simulink model "PV_Array_Application_DC_converor"  (Simulink 7.5)
settings: Solver=ode5  StartTime=0.0  StopTime=10.0  FixedStep=0.00001  RelTol=1e-3
libraries: powerlib x9, simulink x6
settings Model: Creator=Leo216  LastModifiedBy=Leo216

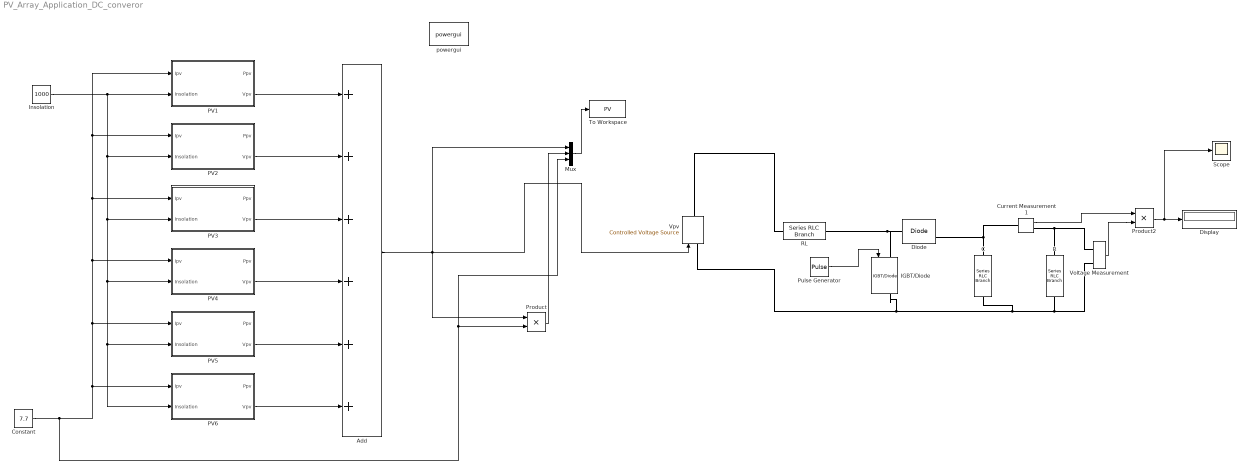
== system PV_Array_Application_DC_converor ==
  Add : Sum  Inputs=++++++  OutDataType=fixdt(1, 16)  OutScaling=2^-10
  C : powerlib/Elements/Series RLC Branch  DialogController=POWERSYS.PowerSysDialog  PhysicalDomain=powersysdomain  SubClassName=unknown  LeftPortType=p1  RightPortType=p1  LConnTagsString=__new0  RConnTagsString=__new0  BranchType=C  Resistance=1  Inductance=1e-3  SetiL0=off  InitialCurrent=0  Capacitance=2000e-6  Setx0=off  InitialVoltage=0  Measurements=None
  Constant : Constant  Value=7.7  OutDataType=fixdt(1, 16)  OutScaling=2^0
  Current Measurement1 : powerlib/Measurements/Current Measurement  DialogController=POWERSYS.PowerSysDialog  SystemSampleTime=-1  PhasorSimulation=off  OutputType=Complex  PSBequivalent=0
  Diode : powerlib/Power Electronics/Diode  DialogController=POWERSYS.PowerSysDialog  SystemSampleTime=-1  Ron=0.001  Lon=0  Vf=0.8  IC=0  UseSnubber=off  Rs=500  Cs=250e-9  Measurements=on
  Display : Display
  IGBT/Diode : powerlib/Power Electronics/IGBT//Diode  DialogController=POWERSYS.PowerSysDialog  SystemSampleTime=-1  Ron=1e-3  Rs=1e5  Cs=inf  Measurements=on
  Insolation : Constant  Value=1000  OutDataType=fixdt(1, 16)  OutScaling=2^0  SampleTime=-1
  Mux : Mux  Inputs=3
  PV1 : Subsystem  mask{Isc=8.4, Voc=39.6/63, Ir=7.7, Vr=31.9/63, Diode=on}
      mask prompts: Isc "Short-circuit current"; Voc "Open-Circuit Voltage"; Ir "Current at Pmax"; Vr "Voltage at Pmax"; Diode "By-pass diode"
      mask init:
      | Ns=round(Voc/0.61);
      | Vt=26e-3
      | G= Isc/1000;
      | Vmpc=Vr/Ns;
      | Vocc=Voc/Ns;
      | Rmpp=Vmpc/Ir;
      | 
      | Rp=100*Vocc/Isc;
      | Vdm=Vocc;
      | 
      | for i=1:10
      |     
      |    Idm=Isc-Ir-Vdm/Rp;
      |    Io=(Isc-Vocc/Rp)/(exp(Vocc/Vt)-1);
      |    Vdm=Vt*log(Idm/Io+1);
      |    Rs=(Vdm-Vmpc)/Ir;
      |    Rd=(Rmpp-Rs)*Rp/(Rp-Rmpp+Rs);
      |    Idm=Vt/Rd;
      |    Rp=Vdm/(Isc-Ir-Idm);
      |    
      | end
      mask Display: image(imread('pv.jpg'))
  PV2 : Subsystem  mask{Isc=8.4, Voc=39.6/63, Ir=7.7, Vr=31.9/63, Diode=on}
      mask prompts: Isc "Short-circuit current"; Voc "Open-Circuit Voltage"; Ir "Current at Pmax"; Vr "Voltage at Pmax"; Diode "By-pass diode"
      mask init: same as PV_Array_Application_DC_converor/PV1
      mask Display: image(imread('pv.jpg'))
  PV3 : Subsystem  mask{Isc=8.4, Voc=39.6/63, Ir=7.7, Vr=31.9/63, Diode=on}
      mask prompts: Isc "Short-circuit current"; Voc "Open-Circuit Voltage"; Ir "Current at Pmax"; Vr "Voltage at Pmax"; Diode "By-pass diode"
      mask init: same as PV_Array_Application_DC_converor/PV1
      mask Display: image(imread('pv.jpg'))
  PV4 : Subsystem  mask{Isc=8.4, Voc=39.6/63, Ir=7.7, Vr=31.9/63, Diode=on}
      mask prompts: Isc "Short-circuit current"; Voc "Open-Circuit Voltage"; Ir "Current at Pmax"; Vr "Voltage at Pmax"; Diode "By-pass diode"
      mask init: same as PV_Array_Application_DC_converor/PV1
      mask Display: image(imread('pv.jpg'))
  PV5 : Subsystem  mask{Isc=8.4, Voc=39.6/63, Ir=7.7, Vr=31.9/63, Diode=on}
      mask prompts: Isc "Short-circuit current"; Voc "Open-Circuit Voltage"; Ir "Current at Pmax"; Vr "Voltage at Pmax"; Diode "By-pass diode"
      mask init: same as PV_Array_Application_DC_converor/PV1
      mask Display: image(imread('pv.jpg'))
  PV6 : Subsystem  mask{Isc=8.4, Voc=39.6/63, Ir=7.7, Vr=31.9/63, Diode=on}
      mask prompts: Isc "Short-circuit current"; Voc "Open-Circuit Voltage"; Ir "Current at Pmax"; Vr "Voltage at Pmax"; Diode "By-pass diode"
      mask init: same as PV_Array_Application_DC_converor/PV1
      mask Display: image(imread('pv.jpg'))
  Product : Product  OutDataType=fixdt(1, 16)  OutScaling=2^0  RndMeth=Zero
  Product2 : Product  OutDataType=fixdt(1, 16)  OutScaling=2^0  RndMeth=Zero
  Pulse Generator : DiscretePulseGenerator  PulseType=Time based  Amplitude=1  Period=.0001  PulseWidth=50  PhaseDelay=0  SampleTime=1
  R : powerlib/Elements/Series RLC Branch  DialogController=POWERSYS.PowerSysDialog  PhysicalDomain=powersysdomain  SubClassName=unknown  LeftPortType=p1  RightPortType=p1  LConnTagsString=__new0  RConnTagsString=__new0  BranchType=R  Resistance=1.576  Inductance=1e-3  SetiL0=off  InitialCurrent=0  Capacitance=1e-6  Setx0=off  InitialVoltage=0  Measurements=None
  RL : powerlib/Elements/Series RLC Branch  DialogController=POWERSYS.PowerSysDialog  PhysicalDomain=powersysdomain  SubClassName=unknown  LeftPortType=p1  RightPortType=p1  LConnTagsString=__new0  RConnTagsString=__new0  BranchType=RL  Resistance=0.005  Inductance=6e-3  SetiL0=off  InitialCurrent=0  Capacitance=1e-6  Setx0=off  InitialVoltage=0  Measurements=None
  Scope : Scope
      settings: YMin=17.075  YMax=17.55
  To Workspace : ToWorkspace  VariableName=PV  SampleTime=-1  SaveFormat=Structure
  Voltage Measurement : powerlib/Measurements/Voltage Measurement  DialogController=POWERSYS.PowerSysDialog  SystemSampleTime=-1  PhasorSimulation=off  OutputType=Complex  PSBequivalent=0
  Vpv : powerlib/Electrical Sources/Controlled Voltage Source  DialogController=POWERSYS.PowerSysDialog  SystemSampleTime=-1  Initialize=on  Source_Type=AC  Amplitude=0  Phase=0  Frequency=0  Measurements=None
  powergui : powerlib/powergui  Priority=1  SystemSampleTime=-1  SimulationMode=Discrete  SampleTime=0.00001  frequency=60  SPID=off  DisableSnubberDevices=off  DisableRonSwitches=off  DisableVfSwitches=off  SwTol=0  Interpol=off  frequencyindice=0  echomessages=off  HookPort=off  DisplayEquations=off  FunctionMessages=off  EnableUseOfTLC=off  x0status=blocks  RestoreLinks=warning  ResistiveCurrentMeasurement=off  Ylog=off  Xlog=on  ShowGrid=off  save=off  variable=ZData  ZoomFFT=off  StartTime=0.0  cycles=1  DisplayStyle=1  FreqAxis=off  MaxFrequency=1000  frequencyindicesteady=1  display=off  methode=off
  wires:
  PV1/2(Vpv) -> Add/1
  PV2/2(Vpv) -> Add/2
  PV3/2(Vpv) -> Add/3
  PV4/2(Vpv) -> Add/4
  PV5/2(Vpv) -> Add/5
  PV6/2(Vpv) -> Add/6
  Insolation/1 -> PV1/2(Insolation), PV5/2(Insolation), PV6/2(Insolation), PV4/2(Insolation), PV3/2(Insolation), PV2/2(Insolation)
  Constant/1 -> PV1/1(Ipv), PV2/1(Ipv), PV3/1(Ipv), PV4/1(Ipv), PV5/1(Ipv), PV6/1(Ipv), Product/2, Mux/3
  Product/1 -> Mux/2
  Mux/1 -> To Workspace/1
  Add/1 -> Mux/1, Product/1, Vpv/1
  Voltage Measurement/1 -> Product2/2
  Product2/1 -> Display/1, Scope/1
  Pulse Generator/1 -> IGBT/Diode/1
  Current Measurement1/1 -> Product2/1
  connections:
  Vpv/RConn1 -- RL/LConn1
  IGBT/Diode/RConn1 -- C/RConn1 -- R/RConn1 -- Voltage Measurement/LConn2 -- Vpv/LConn1
  Voltage Measurement/LConn1 -- R/LConn1 -- Current Measurement1/RConn1
  RL/RConn1 -- Diode/LConn1 -- IGBT/Diode/LConn1
  Current Measurement1/LConn1 -- C/LConn1 -- Diode/RConn1

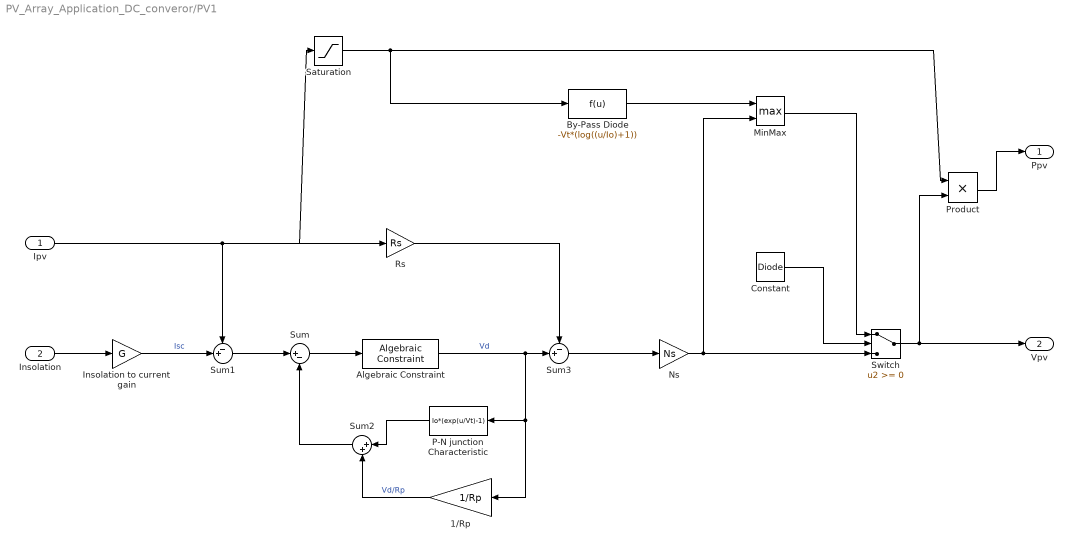
== system PV_Array_Application_DC_converor/PV1 ==
  Ipv : Inport  OutDataType=fixdt(1, 16)  OutScaling=2^0
  Insolation : Inport  Port=2  OutDataType=fixdt(1, 16)  OutScaling=2^0
  1/Rp : Gain  Gain=1/Rp  ParameterDataType=fixdt(1, 16)  ParameterScaling=2^0  OutDataType=fixdt(1, 16)  OutScaling=2^0
  Algebraic Constraint : simulink/Math Operations/Algebraic Constraint  SystemSampleTime=-1  z0=0.5
  By-Pass Diode : Fcn  Expr=-Vt*(log((u/Io)+1))
  Constant : Constant  Value=Diode  OutDataType=fixdt(1, 16)  OutScaling=2^0  SampleTime=-1
  Insolation to current gain : Gain  Gain=G  ParameterDataType=fixdt(1, 16)  ParameterScaling=2^0  OutDataType=fixdt(1, 16)  OutScaling=2^0
  MinMax : MinMax  Function=max  Inputs=2  OutDataType=fixdt(1, 16)  OutScaling=2^0
  Ns : Gain  Gain=Ns  ParameterDataType=fixdt(1, 16)  ParameterScaling=2^0  OutDataType=fixdt(1, 16)  OutScaling=2^0
  P-N junction Characteristic : Fcn  Expr=Io*(exp(u/Vt)-1)
  Product : Product  OutDataType=fixdt(1, 16)  OutScaling=2^0  RndMeth=Zero
  Rs : Gain  Gain=Rs  ParameterDataType=fixdt(1, 16)  ParameterScaling=2^0  OutDataType=fixdt(1, 16)  OutScaling=2^0
  Saturation : Saturate  OutDataType=fixdt(1, 16)  OutScaling=2^0
  Sum : Sum  Inputs=|+-  OutDataType=fixdt(1, 16)  OutScaling=2^0
  Sum1 : Sum  Inputs=-+|  OutDataType=fixdt(1, 16)  OutScaling=2^0
  Sum2 : Sum  Inputs=|++  OutDataType=fixdt(1, 16)  OutScaling=2^0
  Sum3 : Sum  Inputs=-+|  OutDataType=fixdt(1, 16)  OutScaling=2^0
  Switch : Switch  OutDataType=fixdt(1, 16)  OutScaling=2^0
  Ppv : Outport  OutDataType=fixdt(1, 16)  OutScaling=2^0
  Vpv : Outport  Port=2  OutDataType=fixdt(1, 16)  OutScaling=2^0
  wires:
  Insolation/1 -> Insolation to current gain/1
  Product/1 -> Ppv/1
  By-Pass Diode/1 -> MinMax/1
  P-N junction Characteristic/1 -> Sum2/1
  Saturation/1 -> Product/1, By-Pass Diode/1
  Switch/1 -> Product/2, Vpv/1
  MinMax/1 -> Switch/1
  Constant/1 -> Switch/2
  Ns/1 -> Switch/3, MinMax/2
  Sum3/1 -> Ns/1
  Rs/1 -> Sum3/1
  Algebraic Constraint/1 -> Sum3/2, 1/Rp/1, P-N junction Characteristic/1  "Vd"
  1/Rp/1 -> Sum2/2  "Vd/Rp"
  Sum2/1 -> Sum/2
  Sum/1 -> Algebraic Constraint/1
  Sum1/1 -> Sum/1
  Insolation to current gain/1 -> Sum1/2  "Isc"
  Ipv/1 -> Sum1/1, Rs/1, Saturation/1

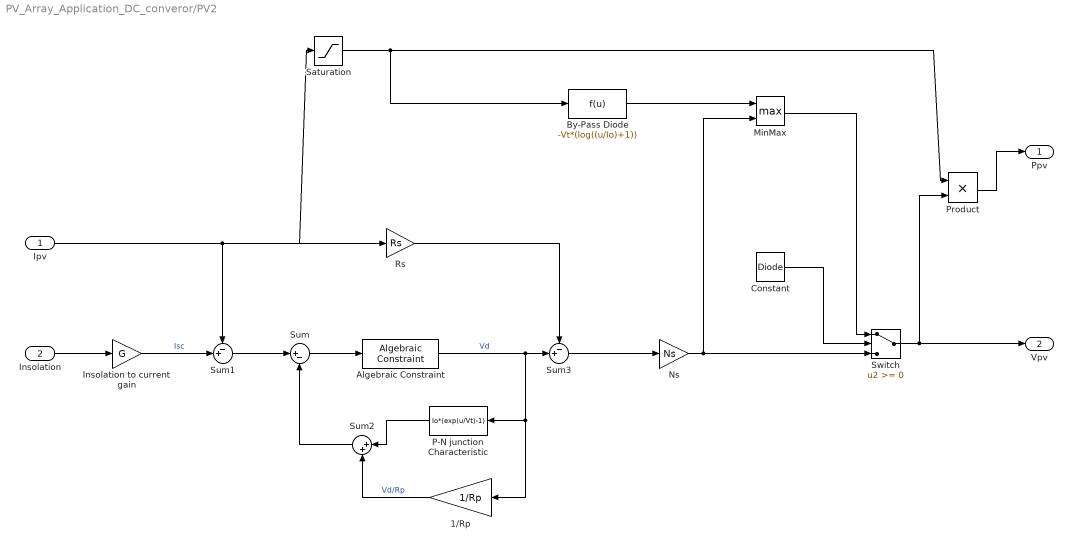
== system PV_Array_Application_DC_converor/PV2 ==
  Ipv : Inport  OutDataType=fixdt(1, 16)  OutScaling=2^0
  Insolation : Inport  Port=2  OutDataType=fixdt(1, 16)  OutScaling=2^0
  1/Rp : Gain  Gain=1/Rp  ParameterDataType=fixdt(1, 16)  ParameterScaling=2^0  OutDataType=fixdt(1, 16)  OutScaling=2^0
  Algebraic Constraint : simulink/Math Operations/Algebraic Constraint  SystemSampleTime=-1  z0=0
  By-Pass Diode : Fcn  Expr=-Vt*(log((u/Io)+1))
  Constant : Constant  Value=Diode  OutDataType=fixdt(1, 16)  OutScaling=2^0  SampleTime=-1
  Insolation to current gain : Gain  Gain=G  ParameterDataType=fixdt(1, 16)  ParameterScaling=2^0  OutDataType=fixdt(1, 16)  OutScaling=2^0
  MinMax : MinMax  Function=max  Inputs=2  OutDataType=fixdt(1, 16)  OutScaling=2^0
  Ns : Gain  Gain=Ns  ParameterDataType=fixdt(1, 16)  ParameterScaling=2^0  OutDataType=fixdt(1, 16)  OutScaling=2^0
  P-N junction Characteristic : Fcn  Expr=Io*(exp(u/Vt)-1)
  Product : Product  OutDataType=fixdt(1, 16)  OutScaling=2^0  RndMeth=Zero
  Rs : Gain  Gain=Rs  ParameterDataType=fixdt(1, 16)  ParameterScaling=2^0  OutDataType=fixdt(1, 16)  OutScaling=2^0
  Saturation : Saturate  OutDataType=fixdt(1, 16)  OutScaling=2^0
  Sum : Sum  Inputs=|+-  OutDataType=fixdt(1, 16)  OutScaling=2^0
  Sum1 : Sum  Inputs=-+|  OutDataType=fixdt(1, 16)  OutScaling=2^0
  Sum2 : Sum  Inputs=|++  OutDataType=fixdt(1, 16)  OutScaling=2^0
  Sum3 : Sum  Inputs=-+|  OutDataType=fixdt(1, 16)  OutScaling=2^0
  Switch : Switch  OutDataType=fixdt(1, 16)  OutScaling=2^0
  Ppv : Outport  OutDataType=fixdt(1, 16)  OutScaling=2^0
  Vpv : Outport  Port=2  OutDataType=fixdt(1, 16)  OutScaling=2^0
  wires:
  Insolation/1 -> Insolation to current gain/1
  Product/1 -> Ppv/1
  By-Pass Diode/1 -> MinMax/1
  P-N junction Characteristic/1 -> Sum2/1
  Saturation/1 -> Product/1, By-Pass Diode/1
  Switch/1 -> Product/2, Vpv/1
  MinMax/1 -> Switch/1
  Constant/1 -> Switch/2
  Ns/1 -> Switch/3, MinMax/2
  Sum3/1 -> Ns/1
  Rs/1 -> Sum3/1
  Algebraic Constraint/1 -> Sum3/2, 1/Rp/1, P-N junction Characteristic/1  "Vd"
  1/Rp/1 -> Sum2/2  "Vd/Rp"
  Sum2/1 -> Sum/2
  Sum/1 -> Algebraic Constraint/1
  Sum1/1 -> Sum/1
  Insolation to current gain/1 -> Sum1/2  "Isc"
  Ipv/1 -> Sum1/1, Rs/1, Saturation/1

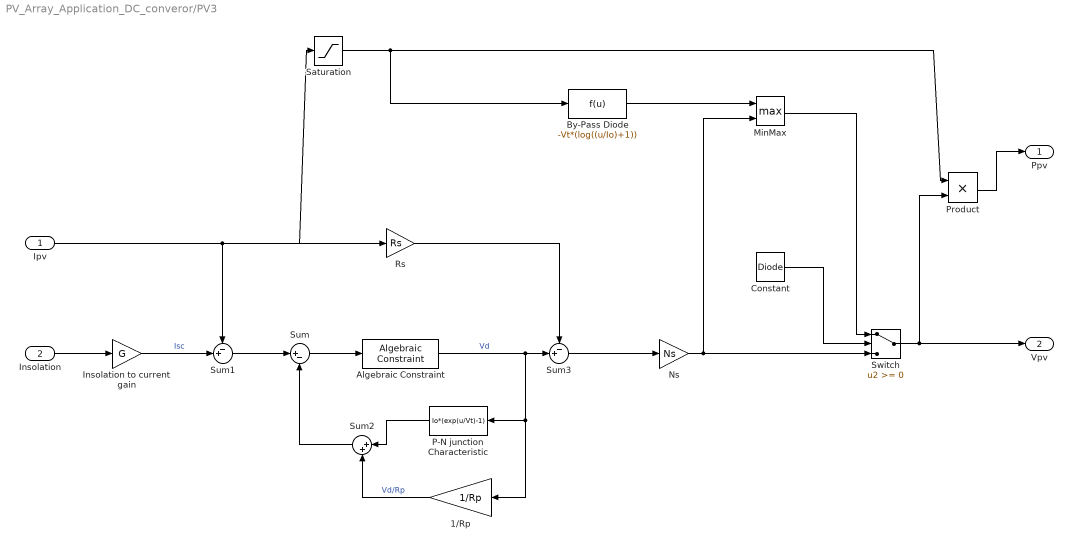
== system PV_Array_Application_DC_converor/PV3 ==
  Ipv : Inport  OutDataType=fixdt(1, 16)  OutScaling=2^0
  Insolation : Inport  Port=2  OutDataType=fixdt(1, 16)  OutScaling=2^0
  1/Rp : Gain  Gain=1/Rp  ParameterDataType=fixdt(1, 16)  ParameterScaling=2^0  OutDataType=fixdt(1, 16)  OutScaling=2^0
  Algebraic Constraint : simulink/Math Operations/Algebraic Constraint  SystemSampleTime=-1  z0=0
  By-Pass Diode : Fcn  Expr=-Vt*(log((u/Io)+1))
  Constant : Constant  Value=Diode  OutDataType=fixdt(1, 16)  OutScaling=2^0  SampleTime=-1
  Insolation to current gain : Gain  Gain=G  ParameterDataType=fixdt(1, 16)  ParameterScaling=2^0  OutDataType=fixdt(1, 16)  OutScaling=2^0
  MinMax : MinMax  Function=max  Inputs=2  OutDataType=fixdt(1, 16)  OutScaling=2^0
  Ns : Gain  Gain=Ns  ParameterDataType=fixdt(1, 16)  ParameterScaling=2^0  OutDataType=fixdt(1, 16)  OutScaling=2^0
  P-N junction Characteristic : Fcn  Expr=Io*(exp(u/Vt)-1)
  Product : Product  OutDataType=fixdt(1, 16)  OutScaling=2^0  RndMeth=Zero
  Rs : Gain  Gain=Rs  ParameterDataType=fixdt(1, 16)  ParameterScaling=2^0  OutDataType=fixdt(1, 16)  OutScaling=2^0
  Saturation : Saturate  OutDataType=fixdt(1, 16)  OutScaling=2^0
  Sum : Sum  Inputs=|+-  OutDataType=fixdt(1, 16)  OutScaling=2^0
  Sum1 : Sum  Inputs=-+|  OutDataType=fixdt(1, 16)  OutScaling=2^0
  Sum2 : Sum  Inputs=|++  OutDataType=fixdt(1, 16)  OutScaling=2^0
  Sum3 : Sum  Inputs=-+|  OutDataType=fixdt(1, 16)  OutScaling=2^0
  Switch : Switch  OutDataType=fixdt(1, 16)  OutScaling=2^0
  Ppv : Outport  OutDataType=fixdt(1, 16)  OutScaling=2^0
  Vpv : Outport  Port=2  OutDataType=fixdt(1, 16)  OutScaling=2^0
  wires:
  Insolation/1 -> Insolation to current gain/1
  Product/1 -> Ppv/1
  By-Pass Diode/1 -> MinMax/1
  P-N junction Characteristic/1 -> Sum2/1
  Saturation/1 -> Product/1, By-Pass Diode/1
  Switch/1 -> Product/2, Vpv/1
  MinMax/1 -> Switch/1
  Constant/1 -> Switch/2
  Ns/1 -> Switch/3, MinMax/2
  Sum3/1 -> Ns/1
  Rs/1 -> Sum3/1
  Algebraic Constraint/1 -> Sum3/2, 1/Rp/1, P-N junction Characteristic/1  "Vd"
  1/Rp/1 -> Sum2/2  "Vd/Rp"
  Sum2/1 -> Sum/2
  Sum/1 -> Algebraic Constraint/1
  Sum1/1 -> Sum/1
  Insolation to current gain/1 -> Sum1/2  "Isc"
  Ipv/1 -> Sum1/1, Rs/1, Saturation/1

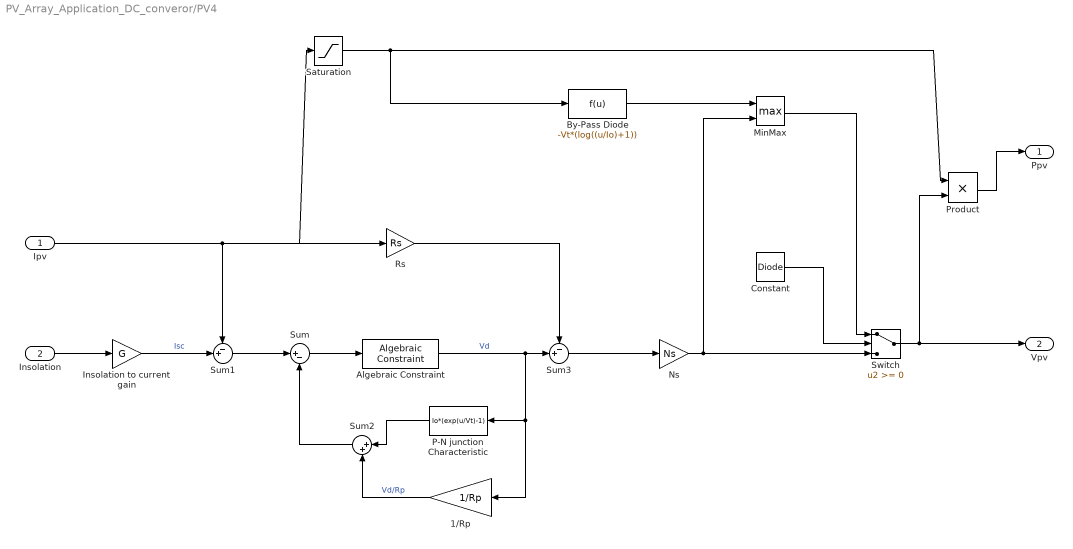
== system PV_Array_Application_DC_converor/PV4 ==
  Ipv : Inport  OutDataType=fixdt(1, 16)  OutScaling=2^0
  Insolation : Inport  Port=2  OutDataType=fixdt(1, 16)  OutScaling=2^0
  1/Rp : Gain  Gain=1/Rp  ParameterDataType=fixdt(1, 16)  ParameterScaling=2^0  OutDataType=fixdt(1, 16)  OutScaling=2^0
  Algebraic Constraint : simulink/Math Operations/Algebraic Constraint  SystemSampleTime=-1  z0=0
  By-Pass Diode : Fcn  Expr=-Vt*(log((u/Io)+1))
  Constant : Constant  Value=Diode  OutDataType=fixdt(1, 16)  OutScaling=2^0
  Insolation to current gain : Gain  Gain=G  ParameterDataType=fixdt(1, 16)  ParameterScaling=2^0  OutDataType=fixdt(1, 16)  OutScaling=2^0
  MinMax : MinMax  Function=max  Inputs=2  OutDataType=fixdt(1, 16)  OutScaling=2^0
  Ns : Gain  Gain=Ns  ParameterDataType=fixdt(1, 16)  ParameterScaling=2^0  OutDataType=fixdt(1, 16)  OutScaling=2^0
  P-N junction Characteristic : Fcn  Expr=Io*(exp(u/Vt)-1)
  Product : Product  OutDataType=fixdt(1, 16)  OutScaling=2^0  RndMeth=Zero
  Rs : Gain  Gain=Rs  ParameterDataType=fixdt(1, 16)  ParameterScaling=2^0  OutDataType=fixdt(1, 16)  OutScaling=2^0
  Saturation : Saturate  OutDataType=fixdt(1, 16)  OutScaling=2^0
  Sum : Sum  Inputs=|+-  OutDataType=fixdt(1, 16)  OutScaling=2^0
  Sum1 : Sum  Inputs=-+|  OutDataType=fixdt(1, 16)  OutScaling=2^0
  Sum2 : Sum  Inputs=|++  OutDataType=fixdt(1, 16)  OutScaling=2^0
  Sum3 : Sum  Inputs=-+|  OutDataType=fixdt(1, 16)  OutScaling=2^0
  Switch : Switch  OutDataType=fixdt(1, 16)  OutScaling=2^0
  Ppv : Outport  OutDataType=fixdt(1, 16)  OutScaling=2^0
  Vpv : Outport  Port=2  OutDataType=fixdt(1, 16)  OutScaling=2^0
  wires:
  Insolation/1 -> Insolation to current gain/1
  Product/1 -> Ppv/1
  By-Pass Diode/1 -> MinMax/1
  P-N junction Characteristic/1 -> Sum2/1
  Saturation/1 -> Product/1, By-Pass Diode/1
  Switch/1 -> Product/2, Vpv/1
  MinMax/1 -> Switch/1
  Constant/1 -> Switch/2
  Ns/1 -> Switch/3, MinMax/2
  Sum3/1 -> Ns/1
  Rs/1 -> Sum3/1
  Algebraic Constraint/1 -> Sum3/2, 1/Rp/1, P-N junction Characteristic/1  "Vd"
  1/Rp/1 -> Sum2/2  "Vd/Rp"
  Sum2/1 -> Sum/2
  Sum/1 -> Algebraic Constraint/1
  Sum1/1 -> Sum/1
  Insolation to current gain/1 -> Sum1/2  "Isc"
  Ipv/1 -> Sum1/1, Rs/1, Saturation/1

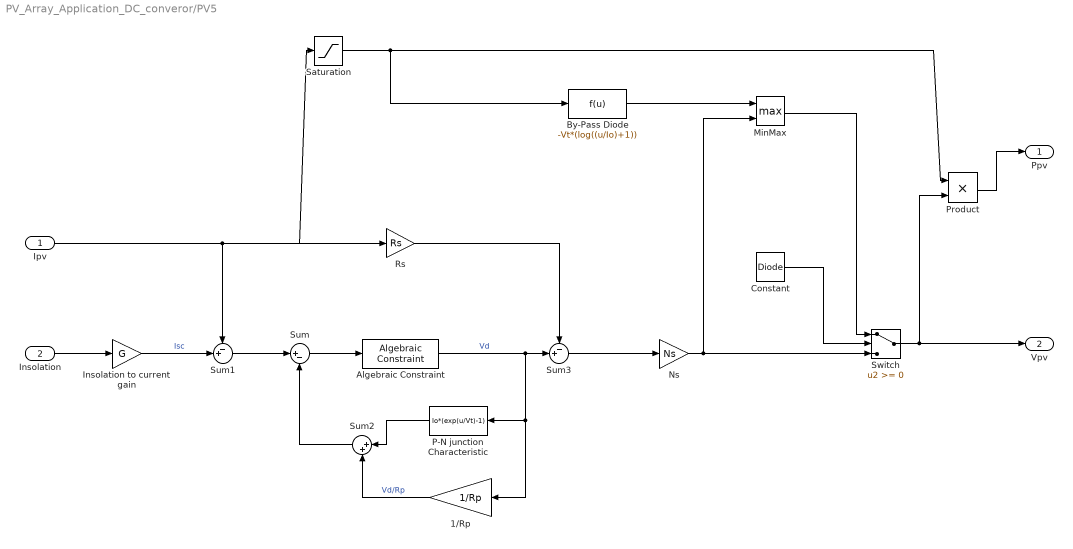
== system PV_Array_Application_DC_converor/PV5 ==
  Ipv : Inport  OutDataType=fixdt(1, 16)  OutScaling=2^0
  Insolation : Inport  Port=2  OutDataType=fixdt(1, 16)  OutScaling=2^0
  1/Rp : Gain  Gain=1/Rp  ParameterDataType=fixdt(1, 16)  ParameterScaling=2^0  OutDataType=fixdt(1, 16)  OutScaling=2^0
  Algebraic Constraint : simulink/Math Operations/Algebraic Constraint  SystemSampleTime=-1  z0=0
  By-Pass Diode : Fcn  Expr=-Vt*(log((u/Io)+1))
  Constant : Constant  Value=Diode  OutDataType=fixdt(1, 16)  OutScaling=2^0
  Insolation to current gain : Gain  Gain=G  ParameterDataType=fixdt(1, 16)  ParameterScaling=2^0  OutDataType=fixdt(1, 16)  OutScaling=2^0
  MinMax : MinMax  Function=max  Inputs=2  OutDataType=fixdt(1, 16)  OutScaling=2^0
  Ns : Gain  Gain=Ns  ParameterDataType=fixdt(1, 16)  ParameterScaling=2^0  OutDataType=fixdt(1, 16)  OutScaling=2^0
  P-N junction Characteristic : Fcn  Expr=Io*(exp(u/Vt)-1)
  Product : Product  OutDataType=fixdt(1, 16)  OutScaling=2^0  RndMeth=Zero
  Rs : Gain  Gain=Rs  ParameterDataType=fixdt(1, 16)  ParameterScaling=2^0  OutDataType=fixdt(1, 16)  OutScaling=2^0
  Saturation : Saturate  OutDataType=fixdt(1, 16)  OutScaling=2^0
  Sum : Sum  Inputs=|+-  OutDataType=fixdt(1, 16)  OutScaling=2^0
  Sum1 : Sum  Inputs=-+|  OutDataType=fixdt(1, 16)  OutScaling=2^0
  Sum2 : Sum  Inputs=|++  OutDataType=fixdt(1, 16)  OutScaling=2^0
  Sum3 : Sum  Inputs=-+|  OutDataType=fixdt(1, 16)  OutScaling=2^0
  Switch : Switch  OutDataType=fixdt(1, 16)  OutScaling=2^0
  Ppv : Outport  OutDataType=fixdt(1, 16)  OutScaling=2^0
  Vpv : Outport  Port=2  OutDataType=fixdt(1, 16)  OutScaling=2^0
  wires:
  Insolation/1 -> Insolation to current gain/1
  Product/1 -> Ppv/1
  By-Pass Diode/1 -> MinMax/1
  P-N junction Characteristic/1 -> Sum2/1
  Saturation/1 -> Product/1, By-Pass Diode/1
  Switch/1 -> Product/2, Vpv/1
  MinMax/1 -> Switch/1
  Constant/1 -> Switch/2
  Ns/1 -> Switch/3, MinMax/2
  Sum3/1 -> Ns/1
  Rs/1 -> Sum3/1
  Algebraic Constraint/1 -> Sum3/2, 1/Rp/1, P-N junction Characteristic/1  "Vd"
  1/Rp/1 -> Sum2/2  "Vd/Rp"
  Sum2/1 -> Sum/2
  Sum/1 -> Algebraic Constraint/1
  Sum1/1 -> Sum/1
  Insolation to current gain/1 -> Sum1/2  "Isc"
  Ipv/1 -> Sum1/1, Rs/1, Saturation/1

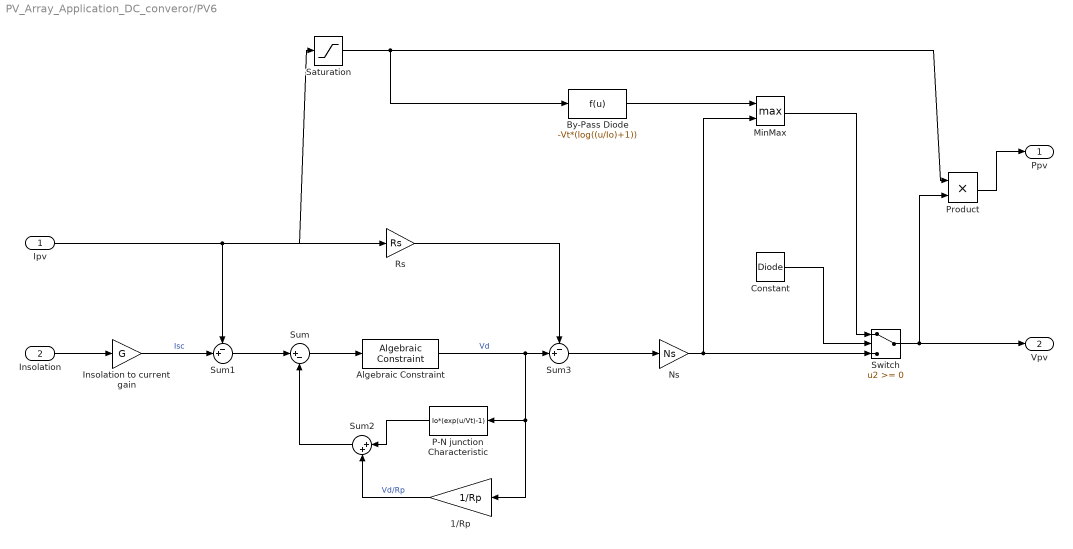
== system PV_Array_Application_DC_converor/PV6 ==
  Ipv : Inport  OutDataType=fixdt(1, 16)  OutScaling=2^0
  Insolation : Inport  Port=2  OutDataType=fixdt(1, 16)  OutScaling=2^0
  1/Rp : Gain  Gain=1/Rp  ParameterDataType=fixdt(1, 16)  ParameterScaling=2^0  OutDataType=fixdt(1, 16)  OutScaling=2^0
  Algebraic Constraint : simulink/Math Operations/Algebraic Constraint  SystemSampleTime=-1  z0=0
  By-Pass Diode : Fcn  Expr=-Vt*(log((u/Io)+1))
  Constant : Constant  Value=Diode  OutDataType=fixdt(1, 16)  OutScaling=2^0
  Insolation to current gain : Gain  Gain=G  ParameterDataType=fixdt(1, 16)  ParameterScaling=2^0  OutDataType=fixdt(1, 16)  OutScaling=2^0
  MinMax : MinMax  Function=max  Inputs=2  OutDataType=fixdt(1, 16)  OutScaling=2^0
  Ns : Gain  Gain=Ns  ParameterDataType=fixdt(1, 16)  ParameterScaling=2^0  OutDataType=fixdt(1, 16)  OutScaling=2^0
  P-N junction Characteristic : Fcn  Expr=Io*(exp(u/Vt)-1)
  Product : Product  OutDataType=fixdt(1, 16)  OutScaling=2^0  RndMeth=Zero
  Rs : Gain  Gain=Rs  ParameterDataType=fixdt(1, 16)  ParameterScaling=2^0  OutDataType=fixdt(1, 16)  OutScaling=2^0
  Saturation : Saturate  OutDataType=fixdt(1, 16)  OutScaling=2^0
  Sum : Sum  Inputs=|+-  OutDataType=fixdt(1, 16)  OutScaling=2^0
  Sum1 : Sum  Inputs=-+|  OutDataType=fixdt(1, 16)  OutScaling=2^0
  Sum2 : Sum  Inputs=|++  OutDataType=fixdt(1, 16)  OutScaling=2^0
  Sum3 : Sum  Inputs=-+|  OutDataType=fixdt(1, 16)  OutScaling=2^0
  Switch : Switch  OutDataType=fixdt(1, 16)  OutScaling=2^0
  Ppv : Outport  OutDataType=fixdt(1, 16)  OutScaling=2^0
  Vpv : Outport  Port=2  OutDataType=fixdt(1, 16)  OutScaling=2^0
  wires:
  Insolation/1 -> Insolation to current gain/1
  Product/1 -> Ppv/1
  By-Pass Diode/1 -> MinMax/1
  P-N junction Characteristic/1 -> Sum2/1
  Saturation/1 -> Product/1, By-Pass Diode/1
  Switch/1 -> Product/2, Vpv/1
  MinMax/1 -> Switch/1
  Constant/1 -> Switch/2
  Ns/1 -> Switch/3, MinMax/2
  Sum3/1 -> Ns/1
  Rs/1 -> Sum3/1
  Algebraic Constraint/1 -> Sum3/2, 1/Rp/1, P-N junction Characteristic/1  "Vd"
  1/Rp/1 -> Sum2/2  "Vd/Rp"
  Sum2/1 -> Sum/2
  Sum/1 -> Algebraic Constraint/1
  Sum1/1 -> Sum/1
  Insolation to current gain/1 -> Sum1/2  "Isc"
  Ipv/1 -> Sum1/1, Rs/1, Saturation/1
